simulink model "Model_PurePursuit"  (R2025b)
settings: Solver=VariableStepAuto  StartTime=0.0  StopTime=150  RelTol=0.01  AbsTol=0.01  EnableMultiTasking=on
undefined symbols (not defined in the file): waypoints, X, Y, Z
libraries: sm_lib x81, nesl_utility x35, slpidlib x2, robotalgslib x1, sharedtransform x1
(part 5 of 5)

== matlab function Model_PurePursuit/RR_climb/MATLAB Function4 ==
  data: t input; q output; mode_cmd input
function q = knee_RL_motion(t, mode_cmd)
% --- Rear Left (RL) Knee Joint Motion Planner ---

% ====================
% Time Nodes
% ====================
T_squat_start = 102;
T_tuck_start  = 146;  % [New] Time to start tucking legs (Preparation)
T_climb_start = 155;  % Time to start actual stair climbing

% ====================
% Phase 0: Wheeled Mode (Idle)
% ====================
if (mode_cmd == 1) || (t < T_squat_start)
    q = 0; 
    return;
end

% ==========================================
% Phase 1: Static Squat Test (102s ~ 130s)
% ==========================================
if t < T_tuck_start
    tau = t - T_squat_start;
    q_stand = 0;
    q_squat = -deg2rad(70);
    T1 = 3;   % Descent time
    T2 = 15;  % Hold time
    T3 = 3;   % Ascent time
    
    if tau < T1
        u = tau / T1;
        q = (1-u)*q_stand + u*q_squat;
    elseif tau < T1 + T2
        q = q_squat;
    elseif tau < T1 + T2 + T3
        u = (tau - (T1 + T2)) / T3;
        q = (1-u)*q_squat + u*q_stand;
    else
        q = q_stand;
    end
    return;
end

% ==========================================
% Phase 2: [New] Tuck Preparation (130s ~ 153s)
% Core Strategy: Retract rear wheels forward to shorten the lever arm
% and prevent tipping over during the wait.
% ==========================================
q_stand = 0;
q_tuck  = deg2rad(-20);  % Tuck angle: Bend knee 20 deg to pull wheels in

if t < T_climb_start
    tau = t - T_tuck_start;
    T_transition = 5.0; % Retract slowly over 5 seconds
    
    if tau < T_transition
        u = tau / T_transition;
        q = (1-u)*q_stand + u*q_tuck;
    else
        % Hold the tucked position, waiting for jump/climb signal
        q = q_tuck; 
    end
    return;
end

% ==========================================
% Phase 3: Stair Climbing Motion (Starts at 153s)
% ==========================================
tau = t - T_climb_start;

% Climbing Parameters
% NOTE: The starting point is now 'q_tuck', not 'q_stand'
q_lift  = deg2rad(-80);  % [Important] High lift: Bend deep to clear the step
q_step  = deg2rad(-20);  % Landing: Slightly bent after mounting step
T_up   = 2.0;            % Time to lift
T_hold = 3.0;            % Time to hold in air
T_down = 2.0;            % Time to lower leg

if tau < T_up
    % 1. Transition: Tuck -> Lift
    u = tau / T_up;
    q = (1-u)*q_tuck + u*q_lift; % Interpolate from Tuck angle
    
elseif tau < (T_up + T_hold)
    % 2. Hold High
    q = q_lift;
    
elseif tau < (T_up + T_hold + T_down)
    % 3. Lower Leg (Landing)
    dt = tau - (T_up + T_hold);
    u = dt / T_down;
    q = (1-u)*q_lift + u*q_step;
    
else
    % 4. Stay on Step
    q = q_step;
end
end

== matlab function Model_PurePursuit/RL/MATLAB Function4 ==
  data: t input; w output
function w = wheel_speed(t)
% ====================
% Parameter Definitions
% ====================
% --- Original Parameters ---
Tsw        = 105;   % Time to start initial acceleration
Tacc       = 2;     % Acceleration duration (0 -> V)
V          = 100;   % Target velocity magnitude 1 (Note: originally labeled as torque)
V2         = 20;    % Target velocity magnitude 2
Tdec_start = 125;   % Time to start deceleration (V -> 0)
Tdec       = 3;     % Deceleration duration
Tpause     = 5;     % Pause duration after stopping
Treacc     = 2;     % Re-acceleration duration (0 -> V2)

% --- New Parameters ---
Thold_V2   = 8;     % Duration to hold V2 (Code says 8s)
Tdec2      = 3;     % Second deceleration duration (V2 -> 0)
Tpause2    = 10;    % Second pause duration (Code says 10s)
Treacc2    = 2;     % Third acceleration duration (0 -> V2)

% ====================
% Time Node Calculation
% (Pre-calculating these improves readability and avoids errors)
% ====================
% Node 1: Time when first acceleration to V2 is complete (End of Phase 6)
T_V2_ready = Tdec_start + Tdec + Tpause + Treacc;

% Node 2: Time when holding V2 ends, start second deceleration
T_dec2_start = T_V2_ready + Thold_V2;

% Node 3: Time when second deceleration to 0 is complete
T_stop2_start = T_dec2_start + Tdec2;

% Node 4: Time when second pause ends, start final acceleration
T_last_acc_start = T_stop2_start + Tpause2;

% Node 5: Time when final acceleration to V2 is complete
T_final_stable = T_last_acc_start + Treacc2;

% ====================
% Logic Control
% ====================
% Phase 1: Not started (Idle)
if t < Tsw
    w = 0;

% Phase 2: Linear Acceleration 0 -> V
elseif t < Tsw + Tacc
    u = (t - Tsw) / Tacc;
    w = u * V;

% Phase 3: Hold V (Constant speed)
elseif t < Tdec_start
    w = V;

% Phase 4: Linear Deceleration V -> 0
elseif t < Tdec_start + Tdec
    u = (t - Tdec_start) / Tdec;
    w = V * (1 - u);

% Phase 5: Stop and Wait (Pause 1)
elseif t < Tdec_start + Tdec + Tpause
    w = 0;

% Phase 6: Re-accelerate 0 -> V2
elseif t < T_V2_ready
    u = (t - (Tdec_start + Tdec + Tpause)) / Treacc;
    w = u * V2;

% --------------------
% New Phases
% --------------------
% Phase 7: Hold V2
elseif t < T_dec2_start
    w = V2;

% Phase 8: Second Deceleration V2 -> 0
elseif t < T_stop2_start
    u = (t - T_dec2_start) / Tdec2;
    w = V2 * (1 - u);

% Phase 9: Second Stop and Wait (Pause 2)
elseif t < T_last_acc_start
    w = 0;

% Phase 10: Final Acceleration 0 -> V2
elseif t < T_final_stable
    u = (t - T_last_acc_start) / Treacc2;
    w = u * V2;

% Phase 11: Hold V2 indefinitely
else
    w = V2;
end
end

== matlab function Model_PurePursuit/RR/MATLAB Function4 ==
  data: t input; w output
function w = wheel_speed(t)
Tsw  = 105;   % initial acceleration start time
Tacc = 2;     % acceleration duration
V    = 100;   % target velocity magnitude(actually it`s torque)
V2=18;% secondary target velocity(torque)

Tdec_start = 125;   % deceleration starting time
Tdec = 3;           % deceleration duration
Tpause = 5;         % pause duration after stopping
Treacc = 2;         % re-accelaration duration

% --------------------
% phase 1: not started
% --------------------
if t < Tsw
    w = 0;

% --------------------
% phase 2: linear acceleration 0->V
% --------------------
elseif t < Tsw + Tacc
    u = (t - Tsw) / Tacc;
    w = u * V;

% --------------------
% phase 3：Hold V
% --------------------
elseif t < Tdec_start
    w = V;

% --------------------
% phase 4: linear deceleration V→0
% --------------------
elseif t < Tdec_start + Tdec
    u = (t - Tdec_start) / Tdec;  % 0→1
    w = V * (1 - u);

% --------------------
% phase 5：stop and wait
% --------------------
elseif t < Tdec_start + Tdec + Tpause
    w = 0;

% --------------------
% phase 6：re-accelerate 0→V2
% --------------------
elseif t < Tdec_start + Tdec + Tpause + Treacc
    u = (t - (Tdec_start + Tdec + Tpause)) / Treacc;
    w = u * V2;

elseif t<Tdec_start + Tdec + Tpause + Treacc+3
    w=V2;
elseif t<Tdec_start + Tdec + Tpause + Treacc+3+2
    u=(t-(Tdec_start + Tdec + Tpause + Treacc+3))/2;
    w=u*V;
% --------------------
% phase 7：hold V
% --------------------
else
    w = V;
end
end

== matlab function Model_PurePursuit/RR/MATLAB Function ==
  data: mode_cmd input; alpha input; tau output; q input; dq input; q_cmd input; is_locked output; q_ref output
function [tau, is_locked, q_ref] = LockJointPD(mode_cmd, alpha, q, dq, q_cmd)
%#codegen
% mode_cmd: 0=Walk(folloew q_cmd), 1=Wheel(lock the present angle )
% alpha   : [0,1] flatten faktor(TransferFcnoutput)，0=walk, 1=leg locked
% q,dq    : joint angle/angular velocity
% q_cmd   : walking/standing angle(rad)

Kp = 1200.0;   % start value
Kd =   20.0;
tau_lim = 300.0;

m = uint8(mode_cmd ~= 0);     % uint8(0/1)
a = double(alpha);

persistent q_hold last_mode
if isempty(q_hold),    q_hold    = q;        end   % double
if isempty(last_mode), last_mode = uint8(0); end   % uint8

% step: 0->1 
if (last_mode == uint8(0)) && (m ~= uint8(0))
    q_hold = q;
end
last_mode = m;

% reference angle
q_ref  = a*q_hold + (1-a)*q_cmd;
dq_ref = 0.0;

% PD
tau = Kp*(q_ref - q) + Kd*(dq_ref - dq);

% 
tau = max(min(tau, tau_lim), -tau_lim);

% 
is_locked = (a > 0.5);     % 
end

== matlab function Model_PurePursuit/FR/MATLAB Function ==
  data: mode_cmd input; alpha input; tau output; q input; dq input; q_cmd input; is_locked output; q_ref output
function [tau, is_locked, q_ref] = LockJointPD(mode_cmd, alpha, q, dq, q_cmd)
%#codegen
% mode_cmd: 0=Walk (track q_cmd), 1=Wheeled (lock current angle)
% alpha   : [0,1] smoothing factor (TransferFcn output), 0=fully walking, 1=fully locked
% q,dq    : joint angle/angular velocity
% q_cmd   : walk/stand target angle (radians)
Kp = 1200.0;   % Starting value, tune per joint
Kd =   20.0;
tau_lim = 300.0;
m = uint8(mode_cmd ~= 0);     % Standardize to uint8(0/1)
a = double(alpha);
persistent q_hold last_mode
if isempty(q_hold),    q_hold    = q;        end   % double
if isempty(last_mode), last_mode = uint8(0); end   % uint8
% Rising edge: 0->1, latch current angle
if (last_mode == uint8(0)) && (m ~= uint8(0))
    q_hold = q;
end
last_mode = m;
% Reference angle: interpolate between "hold angle" and "target angle"
q_ref  = a*q_hold + (1-a)*q_cmd;
dq_ref = 0.0;
% PD
tau = Kp*(q_ref - q) + Kd*(dq_ref - dq);
% Saturation
tau = max(min(tau, tau_lim), -tau_lim);
% Debug flag: is leg lock dominant
is_locked = (a > 0.5);     % Can also output m==1
end

== matlab function Model_PurePursuit/FR/MATLAB Function1 ==
  data: mode_cmd input; alpha input; tau output; q input; dq input; q_cmd input; is_locked output; q_ref output
function [tau, is_locked, q_ref] = LockJointPD(mode_cmd, alpha, q, dq, q_cmd)
%#codegen
% mode_cmd: 0=Walk (track q_cmd), 1=Wheeled (lock current angle)
% alpha   : [0,1] smoothing factor (TransferFcn output), 0=fully walking, 1=fully locked
% q,dq    : joint angle/angular velocity
% q_cmd   : walk/stand target angle (radians)
Kp = 1200.0;   % Starting value, tune per joint
Kd =   20.0;
tau_lim = 300.0;
m = uint8(mode_cmd ~= 0);     % Standardize to uint8(0/1)
a = double(alpha);
persistent q_hold last_mode
if isempty(q_hold),    q_hold    = q;        end   % double
if isempty(last_mode), last_mode = uint8(0); end   % uint8
% Rising edge: 0->1, latch current angle
if (last_mode == uint8(0)) && (m ~= uint8(0))
    q_hold = q;
end
last_mode = m;
% Reference angle: interpolate between "hold angle" and "target angle"
q_ref  = a*q_hold + (1-a)*q_cmd;
dq_ref = 0.0;
% PD
tau = Kp*(q_ref - q) + Kd*(dq_ref - dq);
% Saturation
tau = max(min(tau, tau_lim), -tau_lim);
% Debug flag: is leg lock dominant
is_locked = (a > 0.5);     % Can also output m==1
end

== matlab function Model_PurePursuit/FL/MATLAB Function ==
  data: mode_cmd input; alpha input; tau output; q input; dq input; q_cmd input; is_locked output; q_ref output
function [tau, is_locked, q_ref] = LockJointPD(mode_cmd, alpha, q, dq, q_cmd)
%#codegen
% mode_cmd: 0=Walk (track q_cmd), 1=Wheeled (lock current angle)
% alpha   : [0,1] smoothing factor (TransferFcn output), 0=fully walking, 1=fully locked
% q,dq    : joint angle/angular velocity
% q_cmd   : walk/stand target angle (radians)
Kp = 1200.0;   % Starting value, tune per joint
Kd =   20.0;
tau_lim = 300.0;
m = uint8(mode_cmd ~= 0);     % Standardize to uint8(0/1)
a = double(alpha);
persistent q_hold last_mode
if isempty(q_hold),    q_hold    = q;        end   % double
if isempty(last_mode), last_mode = uint8(0); end   % uint8
% Rising edge: 0->1, latch current angle
if (last_mode == uint8(0)) && (m ~= uint8(0))
    q_hold = q;
end
last_mode = m;
% Reference angle: interpolate between "hold angle" and "target angle"
q_ref  = a*q_hold + (1-a)*q_cmd;
dq_ref = 0.0;
% PD
tau = Kp*(q_ref - q) + Kd*(dq_ref - dq);
% Saturation
tau = max(min(tau, tau_lim), -tau_lim);
% Debug flag: is leg lock dominant
is_locked = (a > 0.5);     % Can also output m==1
end

== matlab function Model_PurePursuit/FL/MATLAB Function1 ==
  data: mode_cmd input; alpha input; tau output; q input; dq input; q_cmd input; is_locked output; q_ref output
function [tau, is_locked, q_ref] = LockJointPD(mode_cmd, alpha, q, dq, q_cmd)
%#codegen
% mode_cmd: 0=Walk (track q_cmd), 1=Wheeled (lock current angle)
% alpha   : [0,1] smoothing factor (TransferFcn output), 0=fully walking, 1=fully locked
% q,dq    : joint angle/angular velocity
% q_cmd   : walk/stand target angle (radians)
Kp = 1200.0;   % Starting value, tune per joint
Kd =   20.0;
tau_lim = 300.0;
m = uint8(mode_cmd ~= 0);     % Standardize to uint8(0/1)
a = double(alpha);
persistent q_hold last_mode
if isempty(q_hold),    q_hold    = q;        end   % double
if isempty(last_mode), last_mode = uint8(0); end   % uint8
% Rising edge: 0->1, latch current angle
if (last_mode == uint8(0)) && (m ~= uint8(0))
    q_hold = q;
end
last_mode = m;
% Reference angle: interpolate between "hold angle" and "target angle"
q_ref  = a*q_hold + (1-a)*q_cmd;
dq_ref = 0.0;
% PD
tau = Kp*(q_ref - q) + Kd*(dq_ref - dq);
% Saturation
tau = max(min(tau, tau_lim), -tau_lim);
% Debug flag: is leg lock dominant
is_locked = (a > 0.5);     % Can also output m==1
end

== matlab function Model_PurePursuit/RL/MATLAB Function ==
  data: mode_cmd input; alpha input; tau output; q input; dq input; q_cmd input; is_locked output; q_ref output
function [tau, is_locked, q_ref] = LockJointPD(mode_cmd, alpha, q, dq, q_cmd)
%#codegen
% mode_cmd: 0=Walk (track q_cmd), 1=Wheeled (lock current angle)
% alpha   : [0,1] smoothing factor (TransferFcn output), 0=fully walking, 1=fully locked
% q,dq    : joint angle/angular velocity
% q_cmd   : walk/stand target angle (radians)
Kp = 1200.0;   % Starting value, tune per joint
Kd =   20.0;
tau_lim = 300.0;
m = uint8(mode_cmd ~= 0);     % Standardize to uint8(0/1)
a = double(alpha);
persistent q_hold last_mode
if isempty(q_hold),    q_hold    = q;        end   % double
if isempty(last_mode), last_mode = uint8(0); end   % uint8
% Rising edge: 0->1, latch current angle
if (last_mode == uint8(0)) && (m ~= uint8(0))
    q_hold = q;
end
last_mode = m;
% Reference angle: interpolate between "hold angle" and "target angle"
q_ref  = a*q_hold + (1-a)*q_cmd;
dq_ref = 0.0;
% PD
tau = Kp*(q_ref - q) + Kd*(dq_ref - dq);
% Saturation
tau = max(min(tau, tau_lim), -tau_lim);
% Debug flag: is leg lock dominant
is_locked = (a > 0.5);     % Can also output m==1
end
